simulink model "dronesmodel"  (R2015b)
settings: Solver=VariableStepAuto  StartTime=0.0  StopTime=100  RelTol=1e-3
values from neighbouring files (symbols this model uses):
  De = 7.7*10^(-6)    (= 7.7e-06)    [mainDrones.m]
  Je = 3*10^(-6)    (= 3e-06)    [mainDrones.m]
  Kb = 0.171    [mainDrones.m]
  Kt = 0.171    [mainDrones.m]
  La = 14.8*10^(-3)    (= 0.0148)    [mainDrones.m]
  Ra = 25.6    [mainDrones.m]
libraries: simulink x2
settings Model: Creator=Kelvin  LastModifiedBy=maxwell

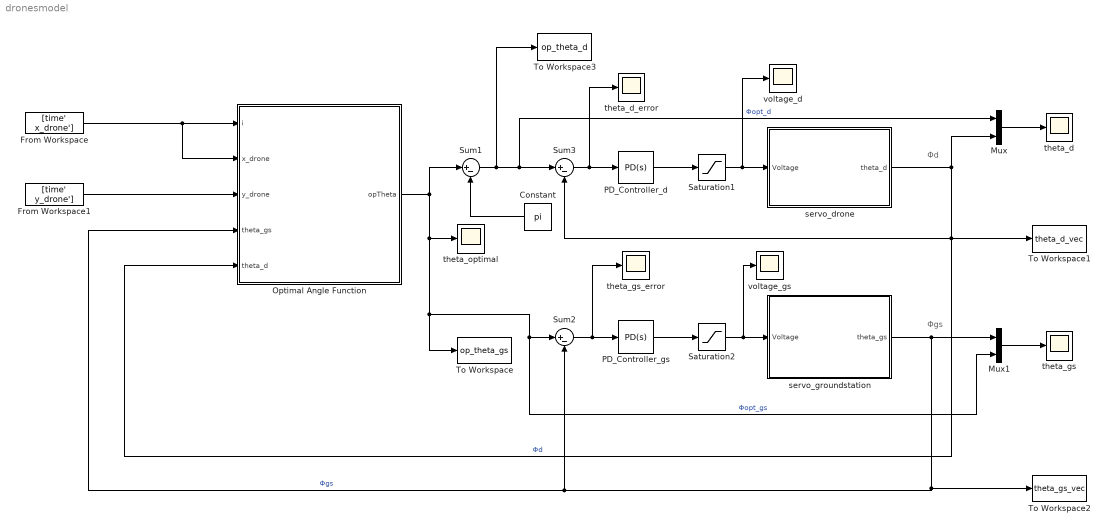
== system dronesmodel ==
  note: Φgs
  note: Φd
  Constant : Constant  Value=pi
  From Workspace : FromWorkspace  VariableName=[time' x_drone']  SampleTime=1
  From Workspace1 : FromWorkspace  VariableName=[time' y_drone']  OutDataTypeStr=double  SampleTime=1
  Mux : Mux  Inputs=2
  Mux1 : Mux  Inputs=2
  "Optimal Angle Function " : MATLAB Function  TreatAsAtomicUnit=on
  PD_Controller_d : simulink/Continuous/PID Controller  Controller=PD  TimeDomain=Continuous-time  SampleTime=-1  IntegratorMethod=Forward Euler  FilterMethod=Forward Euler  Form=Parallel  UseFilter=on  ControllerParametersSource=internal  P=739.414726834109  I=0.0172882676140403  D=150.790271020884  N=52.8940738192282  InitialConditionSource=internal  InitialConditionForIntegrator=0  InitialConditionForFilter=0  ExternalReset=none  LimitOutput=off  UpperSaturationLimit=inf  LowerSaturationLimit=-inf  LinearizeAsGain=on  AntiWindupMode=none  Kb=1  TrackingMode=off  Kt=1  PParamMin=[]  PParamMax=[]  IParamMin=[]  IParamMax=[]  DParamMin=[]  DParamMax=[]  NParamMin=[]  NParamMax=[]  KbParamMin=[]  KbParamMax=[]  KtParamMin=[]  KtParamMax=[]  POutMin=[]  POutMax=[]  IOutMin=[]  IOutMax=[]  DOutMin=[]  DOutMax=[]  NOutMin=[]  NOutMax=[]  KbOutMin=[]  KbOutMax=[]  KtOutMin=[]  KtOutMax=[]  IntegratorOutMin=[]  IntegratorOutMax=[]  FilterOutMin=[]  FilterOutMax=[]  SumOutMin=[]  SumOutMax=[]  SumI1OutMin=[]  SumI1OutMax=[]  SumI2OutMin=[]  SumI2OutMax=[]  SumI3OutMin=[]  SumI3OutMax=[]  SumDOutMin=[]  SumDOutMax=[]  SaturationOutMin=[]  SaturationOutMax=[]  IntegratorContinuousStateAttributes=''  IntegratorStateMustResolveToSignalObject=off  IntegratorRTWStateStorageClass=Auto  FilterContinuousStateAttributes=''  FilterStateMustResolveToSignalObject=off  FilterRTWStateStorageClass=Auto  DifferentiatorICPrevScaledInput=0  DifferentiatorOutMin=[]  DifferentiatorOutMax=[]
  PD_Controller_gs : simulink/Continuous/PID Controller  Controller=PD  TimeDomain=Continuous-time  SampleTime=-1  IntegratorMethod=Forward Euler  FilterMethod=Forward Euler  Form=Parallel  UseFilter=on  ControllerParametersSource=internal  P=739.414726834109  I=0.0172882676140403  D=150.790271020884  N=52.8940738192282  InitialConditionSource=internal  InitialConditionForIntegrator=0  InitialConditionForFilter=0  ExternalReset=none  LimitOutput=off  UpperSaturationLimit=inf  LowerSaturationLimit=-inf  LinearizeAsGain=on  AntiWindupMode=none  Kb=1  TrackingMode=off  Kt=1  PParamMin=[]  PParamMax=[]  IParamMin=[]  IParamMax=[]  DParamMin=[]  DParamMax=[]  NParamMin=[]  NParamMax=[]  KbParamMin=[]  KbParamMax=[]  KtParamMin=[]  KtParamMax=[]  POutMin=[]  POutMax=[]  IOutMin=[]  IOutMax=[]  DOutMin=[]  DOutMax=[]  NOutMin=[]  NOutMax=[]  KbOutMin=[]  KbOutMax=[]  KtOutMin=[]  KtOutMax=[]  IntegratorOutMin=[]  IntegratorOutMax=[]  FilterOutMin=[]  FilterOutMax=[]  SumOutMin=[]  SumOutMax=[]  SumI1OutMin=[]  SumI1OutMax=[]  SumI2OutMin=[]  SumI2OutMax=[]  SumI3OutMin=[]  SumI3OutMax=[]  SumDOutMin=[]  SumDOutMax=[]  SaturationOutMin=[]  SaturationOutMax=[]  IntegratorContinuousStateAttributes=''  IntegratorStateMustResolveToSignalObject=off  IntegratorRTWStateStorageClass=Auto  FilterContinuousStateAttributes=''  FilterStateMustResolveToSignalObject=off  FilterRTWStateStorageClass=Auto  DifferentiatorICPrevScaledInput=0  DifferentiatorOutMin=[]  DifferentiatorOutMax=[]
  Saturation1 : Saturate  UpperLimit=10  LowerLimit=-10
  Saturation2 : Saturate  UpperLimit=10  LowerLimit=-10
  Sum1 : Sum  Inputs=|+-
  Sum2 : Sum  Inputs=|+-
  Sum3 : Sum  Inputs=|+-
  To Workspace : ToWorkspace  VariableName=op_theta_gs  SaveFormat=Timeseries  SampleTime=-1
  To Workspace1 : ToWorkspace  VariableName=theta_d_vec  SaveFormat=Timeseries  SampleTime=-1
  To Workspace2 : ToWorkspace  VariableName=theta_gs_vec  SaveFormat=Timeseries  SampleTime=-1
  To Workspace3 : ToWorkspace  VariableName=op_theta_d  SaveFormat=Timeseries  SampleTime=-1
  servo_drone : Subsystem
  servo_groundstation : Subsystem
  theta_d : Scope
  theta_d_error : Scope
  theta_gs : Scope
  theta_gs_error : Scope
  theta_optimal : Scope
  voltage_d : Scope
  voltage_gs : Scope
  wires:
  From Workspace1/1 -> "Optimal Angle Function "/3(y_drone)
  Constant/1 -> Sum1/2
  "Optimal Angle Function "/1(opTheta) -> Sum1/1, Mux1/2, Sum2/1, To Workspace/1, theta_optimal/1  "Φopt_gs"
  PD_Controller_d/1 -> Saturation1/1
  PD_Controller_gs/1 -> Saturation2/1
  Saturation2/1 -> voltage_gs/1, servo_groundstation/1(Voltage)
  Saturation1/1 -> voltage_d/1, servo_drone/1(Voltage)
  servo_drone/1(theta_d) -> Mux/2, To Workspace1/1, "Optimal Angle Function "/5(theta_d), Sum3/2  "Φd"
  servo_groundstation/1(theta_gs) -> Sum2/2, "Optimal Angle Function "/4(theta_gs), To Workspace2/1, Mux1/1  "Φgs"
  Sum3/1 -> theta_d_error/1, PD_Controller_d/1
  Sum1/1 -> Mux/1, Sum3/1, To Workspace3/1  "Φopt_d"
  Sum2/1 -> theta_gs_error/1, PD_Controller_gs/1
  From Workspace/1 -> "Optimal Angle Function "/1(i), "Optimal Angle Function "/2(x_drone)
  Mux/1 -> theta_d/1
  Mux1/1 -> theta_gs/1

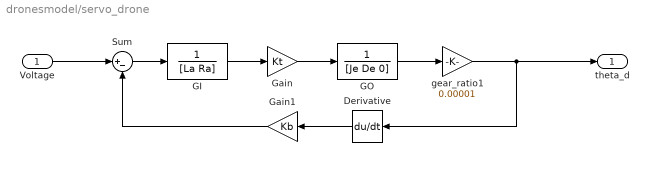
== system dronesmodel/servo_drone ==
  Voltage : Inport
  Derivative : Derivative
  GI : TransferFcn  Denominator=[La Ra]
  GO : TransferFcn  Denominator=[Je De 0]
  Gain : Gain  Gain=Kt
  Gain1 : Gain  Gain=Kb
  Sum : Sum  Inputs=|+-
  "gear_ratio1 " : Gain  Gain=0.00001
  theta_d : Outport
  wires:
  GO/1 -> "gear_ratio1 "/1
  Derivative/1 -> Gain1/1
  Sum/1 -> GI/1
  GI/1 -> Gain/1
  Gain1/1 -> Sum/2
  Gain/1 -> GO/1
  "gear_ratio1 "/1 -> theta_d/1, Derivative/1
  Voltage/1 -> Sum/1

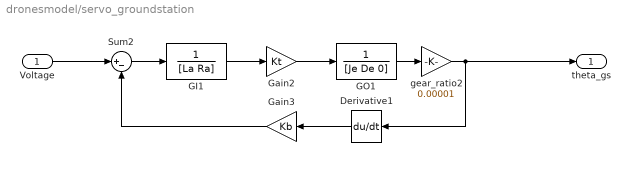
== system dronesmodel/servo_groundstation ==
  Voltage : Inport
  Derivative1 : Derivative
  GI1 : TransferFcn  Denominator=[La Ra]
  GO1 : TransferFcn  Denominator=[Je De 0]
  Gain2 : Gain  Gain=Kt
  Gain3 : Gain  Gain=Kb
  Sum2 : Sum  Inputs=|+-
  gear_ratio2 : Gain  Gain=0.00001
  theta_gs : Outport
  wires:
  GI1/1 -> Gain2/1
  Gain2/1 -> GO1/1
  Derivative1/1 -> Gain3/1
  Gain3/1 -> Sum2/2
  Sum2/1 -> GI1/1
  Voltage/1 -> Sum2/1
  gear_ratio2/1 -> theta_gs/1, Derivative1/1
  GO1/1 -> gear_ratio2/1

== matlab function dronesmodel/Optimal Angle Function  ==
  data: i input; opTheta output; x_drone input; y_drone input; theta_gs input; theta_d input
function opTheta   = funcDronessim(i,x_drone,y_drone,theta_gs,theta_d)
% put here the description of the function
% put here the description of the function
% put here the description of the function
% put here the description of the function

    % Ground station position
    x_gs = 10;                  % The position X of the GROUND STATION 
    y_gs = 0;                   % The position Y of the GROUND STATION     

    % LOS distance vector construction
    if (theta_gs) < 0
        theta_gs = theta_gs + 2*pi;
    end
    if (theta_d) < 0 
        theta_d = theta_d + 2*pi;
    end

    %% Theta error calculations: ALPHA
    % Optimal angles
    if y_drone > y_gs
        opt_theta_gs = atan2(y_drone-y_gs,x_drone-x_gs);
        opt_theta_d = pi + opt_theta_gs;
    else
        opt_theta_d = atan2(y_gs-y_drone,x_gs-x_drone);
        opt_theta_gs = pi + opt_theta_d;
    end

    % Error angles
    alpha_gs = abs(theta_gs - opt_theta_gs);
    alpha_d = abs(theta_d - opt_theta_d);

    if alpha_gs > pi
        alpha_gs = 2*pi - alpha_gs;
    end
    if alpha_d > pi
        alpha_d = 2*pi - alpha_d;
    end
    
    % Optimal angle that we OUTPUT
    opTheta = atan2(y_drone-y_gs,x_drone-x_gs);
    
    %% Ground Station definition (I dont think we need this)
    % Azimuthal angle: of the GROUND STATION FRAME [-pi:pi]. 0 = pointing along
    % X axis
    %%% input to function: theta_gs
    
    % POINTING ANTENNA GS FRAME
%     x_start_gs = x_gs;
%     y_start_gs = y_gs;
%     x_end_gs = x_gs + x_gs/5*cos(theta_gs);
%     y_end_gs = y_gs + x_gs/5*sin(theta_gs);
%     
%     %% Drone definition
%     % Angle of rotation the GROUND STATION FRAME with to the X world
%     %%% input to function: theta_d
%     % POINTING ANTENNA DRONE FRAME
%     x_start_d = x_drone;
%     y_start_d = y_drone; 
%     x_end_d = x_drone + y_drone/5*cos(theta_d);
%     y_end_d = y_drone + y_drone/5*sin(theta_d);
%  
%     %% Calculation
%     alpha_d  = 0;
%     alpha_gs = 0;
%     [alpha_d,alpha_gs] = LOS_angles(x_drone,y_drone,theta_d,x_gs,y_gs,theta_gs);
%     
%     GSgain = 0;
%     Dgain = 0;
%     angle3db_gs = 0;
%     angle3db_d = 0;
%     [GSgain,angle3db_gs] = GSantenna(alpha_gs,0);
%     [Dgain,angle3db_d] = GSantenna(alpha_d,0);
    
end
